simulink model "Model_tan"  (R2017a)
settings: Solver=ode23tb  StartTime=0.0  StopTime=0.3  FixedStep=2e-5  MaxStep=1e-5  RelTol=1e-5  AbsTol=1e-3  EnableMultiTasking=on
values from neighbouring files (symbols this model uses):
  Bs = 1    [Parameters.m]    (also in matlab_Kad.mat)
  L = 0.001    [matlab_Kad.mat]
  Lsr = 0.20106192983    [matlab_Kad.mat]
  omega = 2*pi*50    (= 314.159265359)    [Parameters.m]    (also in matlab_Kad.mat)
  r = 5000    [Parameters.m]    (also in matlab_Kad.mat)
  R0 = 0.225000000000000    (= 0.225)    [Parameters.m]    (also in matlab_Kad.mat)
  S = h*(d1-d2)/2    (= 0.0001875)    [Calc_hysteresis.m]    (also in Parameters.m = 0.000425; matlab_Kad.mat = 0.000425)
  w1 = 1    [Calc_hysteresis.m]    (also in Parameters.m; matlab_Kad.mat)
  w2 = 10    [Calc_hysteresis.m]    (also in Parameters.m = 120; matlab_Kad.mat = 120)
libraries: powerlib x4, simulink x2
settings Model: Creator=Андрей  LastModifiedBy=Aleksey
settings DataIOCC: LimitDataPoints=on  SaveFormat=Array
settings OptimizationCC: LifeSpan=inf
settings DebuggingCC: SolverPrmCheckMsg=warning  SFUnexpectedBacktrackingDiag=warning  SFNoUnconditionalDefaultTransitionDiag=warning  SFExecutionAtInitializationDiag=none
settings HardwareCC: ProdBitPerPointer=32  ProdBitPerSizeT=32  ProdBitPerPtrDiffT=32  ProdLargestAtomicFloat=None  ProdIntDivRoundTo=Undefined  ProdEndianess=Unspecified  ProdWordSize=32  ProdHWDeviceType=32-bit Generic
settings ModelReferenceCC: PropagateSignalLabelsOutOfModel=off
settings GRTTargetCC: TargetLangStandard=C89/C90 (ANSI)  GeneratePreprocessorConditionals=Disable all
settings ConfigComp: CovMetricSettings=dw  CovHtmlReporting=on  CovSaveCumulativeToWorkspaceVar=on  CovSaveSingleToWorkspaceVar=on  CovExternalEMLEnable=off  CovSFcnEnable=off

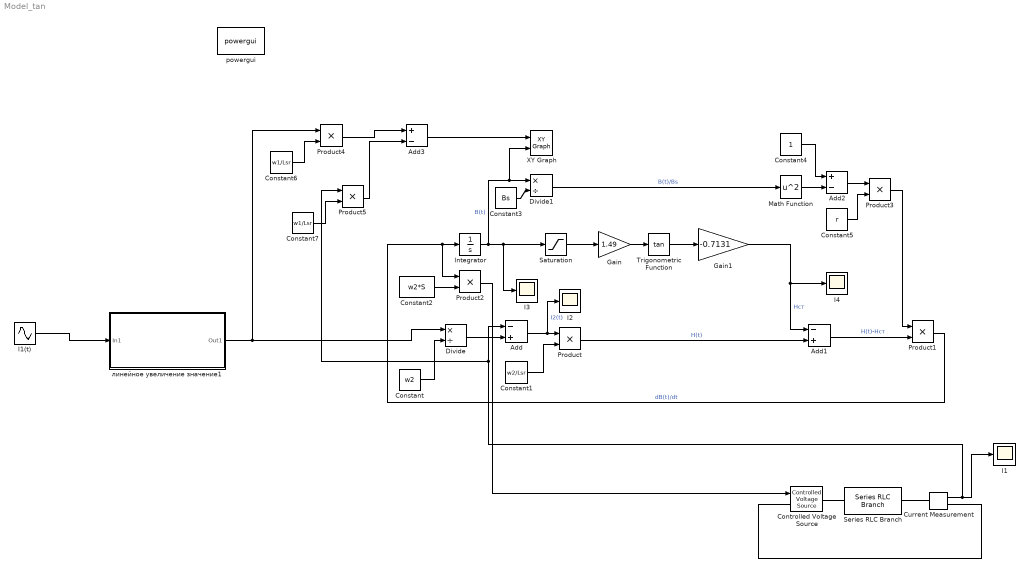
== system Model_tan ==
  Add : Sum  Inputs=-+
  Add1 : Sum  Inputs=-+
  Add2 : Sum  Inputs=+-
  Add3 : Sum  Inputs=+-
  Constant : Constant  Value=w2
  Constant1 : Constant  Value=w2/Lsr
  Constant2 : Constant  Value=w2*S
  Constant3 : Constant  Value=Bs
  Constant4 : Constant
  Constant5 : Constant  Value=r
  Constant6 : Constant  Value=w1/Lsr
  Constant7 : Constant  Value=w1/Lsr
  Controlled Voltage Source : powerlib/Electrical Sources/Controlled Voltage Source  Initialize=on  Source_Type=AC  Amplitude=0  Phase=0  Frequency=0  Measurements=None
  Current Measurement : powerlib/Measurements/Current Measurement  PhasorSimulation=off  OutputType=Complex  PSBequivalent=0
  Divide : Product  Inputs=*/
  Divide1 : Product  Inputs=*/
  Gain : Gain  Gain=1.49
  Gain1 : Gain  Gain=-0.7131
  I{1..4} (4 alike) : Scope
  I1(t) : Sin  Amplitude=9000  Frequency=omega  SampleTime=0
  Integrator : Integrator
  Math Function : Math  Operator=square  SaturateOnIntegerOverflow=on
  Product{,1..5} (6 alike) : Product
  Saturation : Saturate  UpperLimit=1  LowerLimit=-1
  Series RLC Branch : powerlib/Elements/Series RLC Branch  LConnTagsString=__new0  RConnTagsString=__new0  BranchType=RL  Resistance=R0  Inductance=L  SetiL0=off  InitialCurrent=0  Capacitance=1e-6  Setx0=off  InitialVoltage=0  Measurements=None
  Trigonometric Function : Trigonometry  Operator=tan
  XY Graph : simulink/Sinks/XY Graph  xmin=-20  xmax=20  ymin=-1.2  ymax=1.2  st=-1
  powergui : powerlib/powergui  Priority=1  SimulationMode=Continuous  SampleTime=2e-5  frequency=50  Iterations=50  frequencyindice=0  Pbase=100e6  ErrMax=1e-4  UnitsV=kV  UnitsW=MW  buscounter=0  FunctionMessages=off  echomessages=off  EnableUseOfTLC=off  CurrentSourceSwitches=off  DisableSnubberDevices=off  DisableRonSwitches=off  DisableVfSwitches=off  DisplayEquations=off  SolverType=Tustin/Backward Euler (TBE)  Interpol=off  ExternalGateDelay=off  methode=off  Ts=100  x0status=blocks  SPID=off  SwTol=0  HookPort=off  RestoreLinks=warning  ResistiveCurrentMeasurement=off  Frange=[0:2:500]  Ylog=off  Xlog=on  ShowGrid=off  save=off  variable=ZData  structure=0  ZoomFFT=off  StartTime=0.0  cycles=1  DisplayStyle=1  fundamental=60  FreqAxis=off  MaxFrequency=1000  frequencyindicesteady=1  RmsSteady=1  display=off
  линейное увеличение значение1 : Subsystem  mask(линейное увеличение значение){t_rosta=0.1}
      mask prompts: t_rosta "время роста с 0 до максимального значения (c)"
      mask DialogControl ParameterGroupVar Prompt: Параметры
  wires:
  Constant/1 -> Divide/2
  Divide/1 -> Add/2
  Add/1 -> Product/1, I2/1  "I2(t)"
  Constant1/1 -> Product/2
  Product/1 -> Add1/2  "H(t)"
  Add1/1 -> Product1/2  "H(t)-Hст"
  Product1/1 -> Product2/1, Integrator/1  "dB(t)/dt"
  Constant2/1 -> Product2/2
  Integrator/1 -> XY Graph/2, Divide1/1, Saturation/1, I3/1  "B(t)"
  Gain1/1 -> I4/1, Add1/1  "Hст"
  Constant3/1 -> Divide1/2
  Divide1/1 -> Math Function/1  "B(t)/Bs"
  Add2/1 -> Product3/1
  Constant5/1 -> Product3/2
  Product3/1 -> Product1/1
  Math Function/1 -> Add2/2
  Constant4/1 -> Add2/1
  Add3/1 -> XY Graph/1
  Constant6/1 -> Product4/2
  Product2/1 -> Controlled Voltage Source/1
  линейное увеличение значение1/1(Out1) -> Divide/1, Product4/1
  I1(t)/1 -> линейное увеличение значение1/1(In1)
  Product4/1 -> Add3/1
  Current Measurement/1 -> Add/1, Product5/1, I1/1
  Constant7/1 -> Product5/2
  Product5/1 -> Add3/2
  Gain/1 -> Trigonometric Function/1
  Trigonometric Function/1 -> Gain1/1
  Saturation/1 -> Gain/1
  connections:
  Current Measurement/RConn1 -- Controlled Voltage Source/LConn1
  Series RLC Branch/RConn1 -- Current Measurement/LConn1
  Series RLC Branch/LConn1 -- Controlled Voltage Source/RConn1

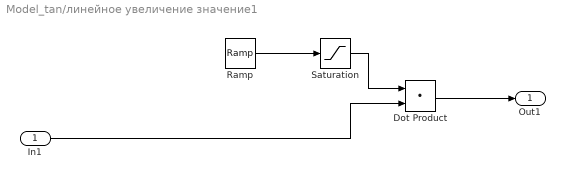
== system Model_tan/линейное увеличение значение1 ==
  In1 : Inport
  Dot Product : DotProduct  InputSameDT=on  OutDataTypeStr=Inherit: Inherit via internal rule
  Ramp : simulink/Sources/Ramp  slope=1/t_rosta  start=0  X0=0
  Saturation : Saturate  UpperLimit=1  LowerLimit=0  ZeroCross=off
  Out1 : Outport
  wires:
  Dot Product/1 -> Out1/1
  Saturation/1 -> Dot Product/1
  Ramp/1 -> Saturation/1
  In1/1 -> Dot Product/2
